simulink model "openLoop"  (R2024a)
settings: Solver=ode45  StartTime=0.0  StopTime=800  RelTol=1e-3
undefined symbols (not defined in the file or in its folder): init, motor
libraries: simulink x1
settings Model: Creator=b_ant  LastModifiedBy=b_ant
settings DataIOCC: SaveFormat=Array

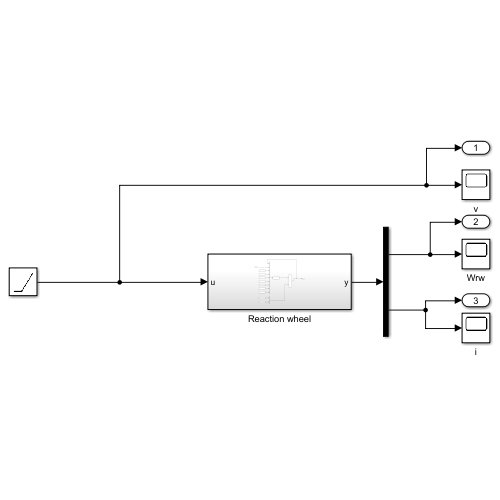
[thumbnail: Simulink's stored preview of the top-level diagram]
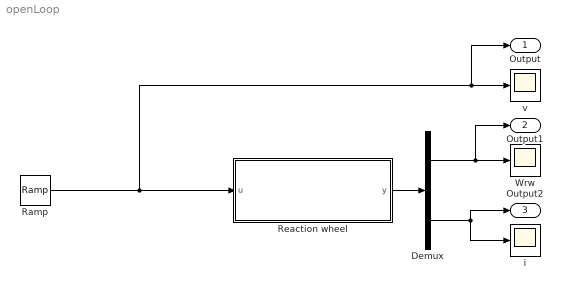
== system openLoop ==
  Demux : Demux  Outputs=2
  Ramp : simulink/Sources/Ramp  slope=0.0300  start=0  InitialOutput=-12
  Reaction wheel : Subsystem
  Wrw : Scope
  i : Scope
  v : Scope
  Output : Outport
  Output1 : Outport  Port=2
  Output2 : Outport  Port=3
  wires:
  Ramp/1 -> Output/1, v/1, Reaction wheel/1(u)
  Reaction wheel/1(y) -> Demux/1
  Demux/1 -> Output1/1, Wrw/1
  Demux/2 -> Output2/1, i/1

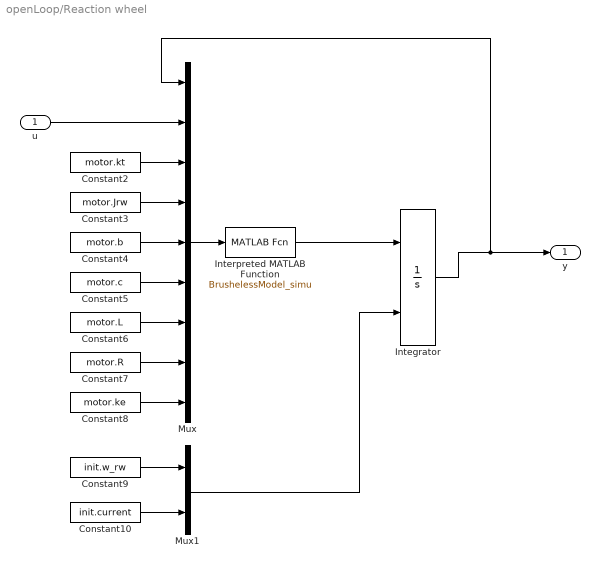
== system openLoop/Reaction wheel ==
  u : Inport
  Constant10 : Constant  Value=init.current
  Constant2 : Constant  Value=motor.kt
  Constant3 : Constant  Value=motor.Jrw
  Constant4 : Constant  Value=motor.b
  Constant5 : Constant  Value=motor.c
  Constant6 : Constant  Value=motor.L
  Constant7 : Constant  Value=motor.R
  Constant8 : Constant  Value=motor.ke
  Constant9 : Constant  Value=init.w_rw
  Integrator : Integrator  InitialConditionSource=external
  Interpreted MATLAB Function : MATLABFcn  MATLABFcn=BrushelessModel_simu  OutputDimensions=2
  Mux : Mux  Inputs=9
  Mux1 : Mux  Inputs=2
  y : Outport
  wires:
  Interpreted MATLAB Function/1 -> Integrator/1
  Constant8/1 -> Mux/9
  Integrator/1 -> Mux/1, y/1
  Constant10/1 -> Mux1/2
  Constant9/1 -> Mux1/1
  Mux/1 -> Interpreted MATLAB Function/1
  Mux1/1 -> Integrator/2
  u/1 -> Mux/2
  Constant2/1 -> Mux/3
  Constant3/1 -> Mux/4
  Constant4/1 -> Mux/5
  Constant5/1 -> Mux/6
  Constant6/1 -> Mux/7
  Constant7/1 -> Mux/8
